simulink model "LQG_Dead_Zone_2"  (R2020a)
settings: Solver=VariableStepAuto  StartTime=0.0  StopTime=500  RelTol=1e-3
values from neighbouring files (symbols this model uses):
  A = stateSpaceModel.A    [System_Control.m]    (also in script2.m)
  B = stateSpaceModel.B    [System_Control.m]    (also in script2.m)
  C = stateSpaceModel.C    [System_Control.m]    (also in script2.m)
  Nbar = Nu+K*Nx    [System_Control.m]    (also in script2.m)
  Ts = stateSpaceModel.Ts    [System_Control.m]    (also in script2.m)
undefined symbols (not defined in the file or in its folder): DiscIntNeverNeededParam, K, M
libraries: simulink x1
settings Model: Creator=Gil  LastModifiedBy=Gil

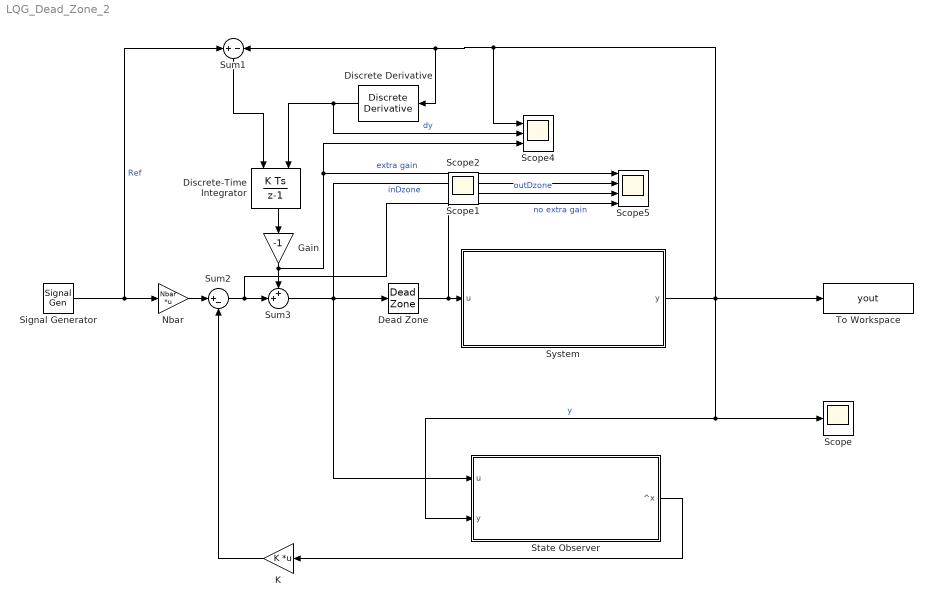
== system LQG_Dead_Zone_2 ==
  Dead Zone : DeadZone  LowerValue=-0.1  UpperValue=0.1  SaturateOnIntegerOverflow=on
  Discrete Derivative : simulink/Discrete/Discrete Derivative  gainval=1.0  ICPrevScaledInput=0.0  OutMin=[]  OutMax=[]  OutDataType=fixdt(1, 16)  OutScaling=2^-10  DoSatur=off
  Discrete-Time Integrator : DiscreteIntegrator  gainval=0.008  ExternalReset=either  SampleTime=Ts  ICPrevOutput=DiscIntNeverNeededParam  ICPrevScaledInput=DiscIntNeverNeededParam
  Gain : Gain  Gain=-1
  K : Gain  Gain=K  Multiplication=Matrix(K*u)
  Nbar : Gain  Gain=Nbar  Multiplication=Matrix(K*u)
  Scope : Scope
  Scope4 : Scope  NumInputPorts=3
  Scope5 : Scope  NumInputPorts=4
  Signal Generator : SignalGenerator  WaveForm=square  Amplitude=5  Frequency=1/50
  State Observer : Subsystem
  Sum1 : Sum  Inputs=+-
  Sum2 : Sum  Inputs=|+-
  Sum3 : Sum  Inputs=++|
  System : Subsystem
  To Workspace : ToWorkspace  VariableName=yout  SaveFormat=Structure With Time  SampleTime=Ts
  Scope1 : Scope
  Scope2 : Scope
  wires:
  K/1 -> Sum2/2
  Sum3/1 -> Scope5/2, State Observer/1(u), Dead Zone/1  "inDzone"
  State Observer/1(^x) -> K/1
  System/1(y) -> To Workspace/1, Scope4/1, Discrete Derivative/1, Sum1/2, State Observer/2(y), Scope/1  "y"
  Signal Generator/1 -> Sum1/1, Nbar/1  "Ref"
  Dead Zone/1 -> Scope5/3, System/1(u)  "outDzone"
  Sum1/1 -> Discrete-Time Integrator/1
  Discrete-Time Integrator/1 -> Gain/1
  Gain/1 -> Sum3/1, Scope4/3, Scope5/1  "extra gain"
  Discrete Derivative/1 -> Discrete-Time Integrator/2, Scope4/2  "dy"
  Nbar/1 -> Sum2/1
  Sum2/1 -> Scope5/4, Sum3/2  "no extra gain"

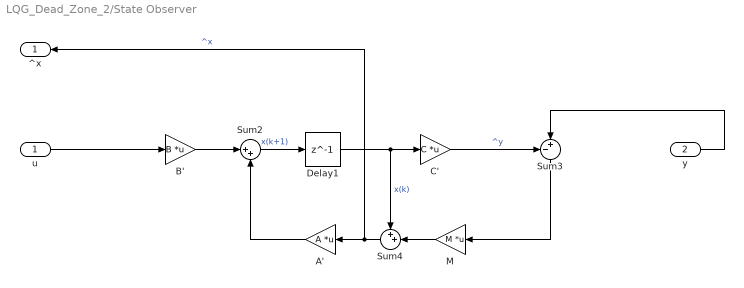
== system LQG_Dead_Zone_2/State Observer ==
  u : Inport
  y : Inport  Port=2
  A' : Gain  Gain=A  Multiplication=Matrix(K*u)
  B' : Gain  Gain=B  Multiplication=Matrix(K*u)
  C' : Gain  Gain=C  Multiplication=Matrix(K*u)
  Delay1 : Delay  DelayLength=1  InitialCondition=0  SampleTime=Ts
  M : Gain  Gain=M  Multiplication=Matrix(K*u)
  Sum2 : Sum  Inputs=|++
  Sum3 : Sum  Inputs=-+|
  Sum4 : Sum  Inputs=++|
  ^x : Outport
  wires:
  Sum4/1 -> ^x/1, A'/1  "^x"
  A'/1 -> Sum2/2
  M/1 -> Sum4/2
  B'/1 -> Sum2/1
  Delay1/1 -> Sum4/1, C'/1  "x(k)"
  C'/1 -> Sum3/1  "^y"
  Sum3/1 -> M/1
  y/1 -> Sum3/2
  Sum2/1 -> Delay1/1  "x(k+1)"
  u/1 -> B'/1

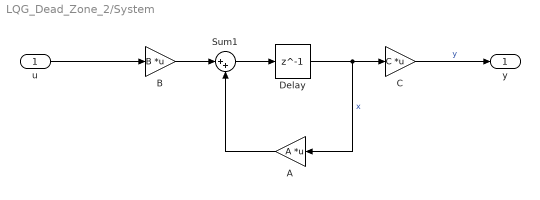
== system LQG_Dead_Zone_2/System ==
  u : Inport
  "A " : Gain  Gain=A  Multiplication=Matrix(K*u)
  B : Gain  Gain=B  Multiplication=Matrix(K*u)
  C : Gain  Gain=C  Multiplication=Matrix(K*u)
  Delay : Delay  DelayLength=1  InitialCondition=0  SampleTime=Ts
  Sum1 : Sum  Inputs=|++
  y : Outport
  wires:
  u/1 -> B/1
  "A "/1 -> Sum1/2
  C/1 -> y/1  "y"
  Delay/1 -> "A "/1, C/1  "x"
  Sum1/1 -> Delay/1
  B/1 -> Sum1/1
